simulink model "chirp_rev_detect"  (R2025b)
settings: Solver=FixedStepAuto  StartTime=0.0  StopTime=25  RelTol=1e-3  EnableMultiTasking=on
libraries: dspfdesign x3
settings Model: Creator=Administrator  LastModifiedBy=padhia
settings SolverCC: AlgebraicLoopSolver=TrustRegion  PositivePriorityOrder=on
settings OptimizationCC: EnhancedBackFolding=on  PassReuseOutputArgsAs=Individual arguments  ZeroExternalMemoryAtStartup=off  ZeroInternalMemoryAtStartup=off  MaxStackSize=200000  OptimizeBlockOrder=speed  DifferentSizesBufferReuse=on  OptimizationCustomize=off  EfficientTunableParamExpr=on
settings DebuggingCC: ParameterTunabilityLossMsg=error  UnconnectedInputMsg=warning  UnconnectedOutputMsg=warning  UnconnectedLineMsg=warning
settings HardwareCC: ProdBitPerPointer=32.0  ProdBitPerSizeT=32.0  ProdBitPerPtrDiffT=32.0  ProdLargestAtomicInteger=Long  ProdLargestAtomicFloat=Double  ProdWordSize=32.0  ProdLongLongMode=on  ProdHWDeviceType=ARM Compatible->ARM Cortex-A (32-bit)
settings ModelReferenceCC: EnableRefExpFcnMdlSchedulingChecks=on
settings RTWCC: SystemTargetFile=ert.tlc  GenCodeOnly=on  TemplateMakefile=ert_default_tmf  RTWVerbose=off  Toolchain=GNU GCC Embedded Linux  BuildConfiguration=Faster Runs  IncludeHyperlinkInReport=on  GPUComputeCapability=3.5  Description=Embedded Coder
settings CodeAppCC: ForceParamTrailComments=on  IgnoreCustomStorageClasses=off  OperatorAnnotations=on  SimulinkDataObjDesc=on  SFDataObjDesc=on  InsertBlockDesc=on
settings ERTTargetCC: InlinedParameterPlacement=Hierarchical  ERTCustomFileTemplate=example_file_process.tlc  DynamicArrayContainerType=coder::array  SupportVariableSizeSignals=on

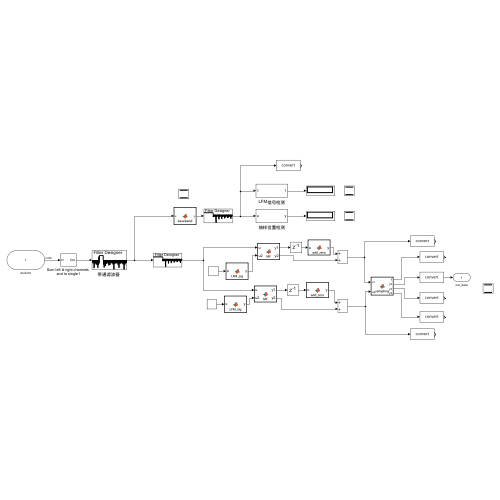
[thumbnail: Simulink's stored preview of the top-level diagram]
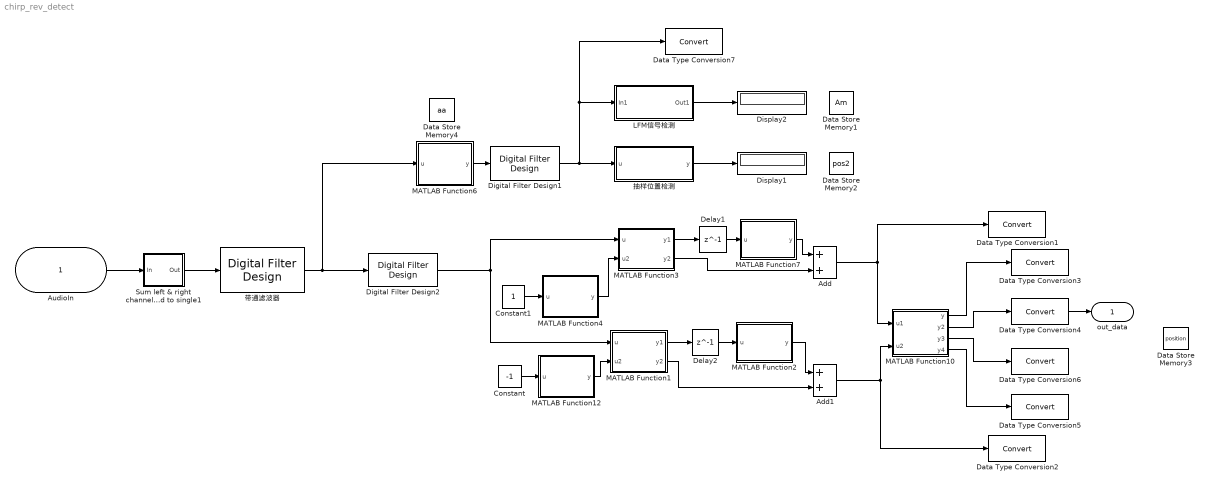
== system chirp_rev_detect ==
  AudioIn : Inport  OutDataTypeStr=int16  PortDimensions=[800 2]  SampleTime=0.1
  Add : Sum
  Add1 : Sum
  Constant : Constant  Value=-1
  Constant1 : Constant
  Data Store Memory1 : DataStoreMemory  DataStoreName=Am  ReadBeforeWriteMsg=warning  WriteAfterWriteMsg=warning  WriteAfterReadMsg=warning  ShowAdditionalParam=off  OutDataTypeStr=double
  Data Store Memory2 : DataStoreMemory  DataStoreName=pos2  ReadBeforeWriteMsg=warning  WriteAfterWriteMsg=warning  WriteAfterReadMsg=warning  ShowAdditionalParam=off  OutDataTypeStr=double
  Data Store Memory3 : DataStoreMemory  DataStoreName=position  ReadBeforeWriteMsg=warning  WriteAfterWriteMsg=warning  WriteAfterReadMsg=warning  ShowAdditionalParam=off  OutDataTypeStr=double
  Data Store Memory4 : DataStoreMemory  DataStoreName=aa  ReadBeforeWriteMsg=warning  WriteAfterWriteMsg=warning  WriteAfterReadMsg=warning  ShowAdditionalParam=off  OutDataTypeStr=double
  Data Type Conversion{1..7} (7 alike) : DataTypeConversion  SaturateOnIntegerOverflow=off  RndMeth=Floor
  Delay1 : Delay  DelayLength=1  InitialCondition=0
  Delay2 : Delay  DelayLength=1  InitialCondition=0
  Digital Filter Design1 : dspfdesign/Digital Filter Design  mwdsp_browser_bugfix_var=off
  Digital Filter Design2 : dspfdesign/Digital Filter Design  mwdsp_browser_bugfix_var=off
  Display1 : Display
  Display2 : Display
  LFM信号检测 : Subsystem
  MATLAB Function1 : MATLAB Function  TreatAsAtomicUnit=on
  MATLAB Function10 : MATLAB Function  TreatAsAtomicUnit=on
  MATLAB Function12 : MATLAB Function  TreatAsAtomicUnit=on
  MATLAB Function2 : MATLAB Function  TreatAsAtomicUnit=on
  MATLAB Function3 : MATLAB Function  TreatAsAtomicUnit=on
  MATLAB Function4 : MATLAB Function  TreatAsAtomicUnit=on
  MATLAB Function6 : MATLAB Function  TreatAsAtomicUnit=on
  MATLAB Function7 : MATLAB Function  TreatAsAtomicUnit=on
  Sum left & right channels and to single1 : Subsystem
  "带通滤波器 " : dspfdesign/Digital Filter Design  mwdsp_browser_bugfix_var=off
  抽样位置检测 : Subsystem
  out_data : Outport
  wires:
  MATLAB Function3/1(y1) -> Delay1/1
  MATLAB Function4/1(y) -> MATLAB Function3/2(u2)
  Digital Filter Design2/1 -> MATLAB Function3/1(u), MATLAB Function1/1(u)
  Add1/1 -> Data Type Conversion2/1, MATLAB Function10/2(u2)
  MATLAB Function10/1(y) -> Data Type Conversion3/1
  MATLAB Function3/2(y2) -> Add/2
  Constant1/1 -> MATLAB Function4/1(u)
  MATLAB Function10/2(y2) -> Data Type Conversion4/1
  Delay2/1 -> MATLAB Function2/1(u)
  MATLAB Function7/1(y) -> Add/1
  Sum left & right channels and to single1/1(Out) -> "带通滤波器 "/1
  MATLAB Function2/1(y) -> Add1/1
  Add/1 -> Data Type Conversion1/1, MATLAB Function10/1(u1)
  MATLAB Function10/3(y3) -> Data Type Conversion6/1
  MATLAB Function1/1(y1) -> Delay2/1
  Constant/1 -> MATLAB Function12/1(u)
  MATLAB Function12/1(y) -> MATLAB Function1/2(u2)
  Delay1/1 -> MATLAB Function7/1(u)
  MATLAB Function1/2(y2) -> Add1/2
  Digital Filter Design1/1 -> 抽样位置检测/1(u), Data Type Conversion7/1, LFM信号检测/1(In1)
  LFM信号检测/1(Out1) -> Display2/1
  "带通滤波器 "/1 -> Digital Filter Design2/1, MATLAB Function6/1(u)
  MATLAB Function6/1(y) -> Digital Filter Design1/1
  MATLAB Function10/4(y4) -> Data Type Conversion5/1
  抽样位置检测/1(y) -> Display1/1
  AudioIn/1 -> Sum left & right channels and to single1/1(In)
  Data Type Conversion4/1 -> out_data/1

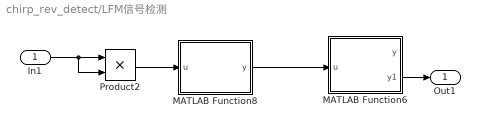
== system chirp_rev_detect/LFM信号检测 ==
  In1 : Inport
  MATLAB Function6 : MATLAB Function  TreatAsAtomicUnit=on
  MATLAB Function8 : MATLAB Function  TreatAsAtomicUnit=on
  Product2 : Product
  Out1 : Outport
  wires:
  Product2/1 -> MATLAB Function8/1(u)
  MATLAB Function8/1(y) -> MATLAB Function6/1(u)
  MATLAB Function6/2(y1) -> Out1/1
  In1/1 -> Product2/2, Product2/1

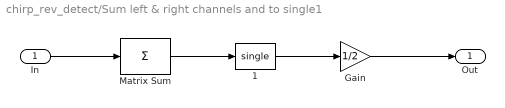
== system chirp_rev_detect/Sum left & right channels and to single1 ==
  In : Inport
  " 1" : DataTypeConversion  OutDataTypeStr=single  SaturateOnIntegerOverflow=off  RndMeth=Floor
  Gain : Gain  Gain=1/2
  Matrix Sum : Sum  Inputs=+  CollapseMode=Specified dimension  CollapseDim=2
  Out : Outport  VectorParamsAs1DForOutWhenUnconnected=off
  wires:
  Gain/1 -> Out/1
  In/1 -> Matrix Sum/1
  Matrix Sum/1 -> " 1"/1
  " 1"/1 -> Gain/1

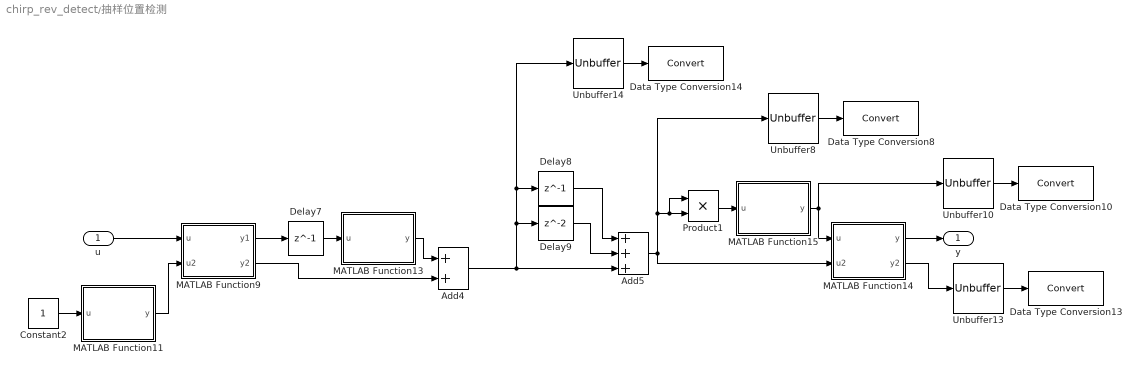
== system chirp_rev_detect/抽样位置检测 ==
  u : Inport
  Add4 : Sum
  Add5 : Sum  Inputs=+++
  Constant2 : Constant
  Data Type Conversion{8,10,13..14} (4 alike) : DataTypeConversion  SaturateOnIntegerOverflow=off  RndMeth=Floor
  Delay7 : Delay  DelayLength=1  InitialCondition=0
  Delay8 : Delay  DelayLength=1  InitialCondition=0
  Delay9 : Delay  InitialCondition=0
  MATLAB Function11 : MATLAB Function  TreatAsAtomicUnit=on
  MATLAB Function13 : MATLAB Function  TreatAsAtomicUnit=on
  MATLAB Function14 : MATLAB Function  TreatAsAtomicUnit=on
  MATLAB Function15 : MATLAB Function  TreatAsAtomicUnit=on
  MATLAB Function9 : MATLAB Function  TreatAsAtomicUnit=on
  Product1 : Product
  Unbuffer{8,10,13..14} (4 alike) : Unbuffer
  y : Outport
  wires:
  Add4/1 -> Unbuffer14/1, Delay8/1, Delay9/1, Add5/3
  MATLAB Function9/2(y2) -> Add4/2
  MATLAB Function11/1(y) -> MATLAB Function9/2(u2)
  Constant2/1 -> MATLAB Function11/1(u)
  Delay7/1 -> MATLAB Function13/1(u)
  MATLAB Function15/1(y) -> Unbuffer10/1, MATLAB Function14/1(u)
  MATLAB Function9/1(y1) -> Delay7/1
  Unbuffer13/1 -> Data Type Conversion13/1
  Delay8/1 -> Add5/1
  MATLAB Function14/2(y2) -> Unbuffer13/1
  Delay9/1 -> Add5/2
  Add5/1 -> MATLAB Function14/2(u2), Unbuffer8/1, Product1/1, Product1/2
  MATLAB Function13/1(y) -> Add4/1
  Unbuffer8/1 -> Data Type Conversion8/1
  Product1/1 -> MATLAB Function15/1(u)
  Unbuffer14/1 -> Data Type Conversion14/1
  Unbuffer10/1 -> Data Type Conversion10/1
  u/1 -> MATLAB Function9/1(u)
  MATLAB Function14/1(y) -> y/1

== matlab function chirp_rev_detect/MATLAB Function12 ==
  data: u input; y output
function y  = LFM_sig(u)
%% miu为1的chrip信号 %%
fs=8000;
T=1e-1;
B=200;                      %信号高频带宽，BT>>1
k=B/T;                      %调频斜率
n=round(T*fs);              %采样点个数
t=linspace(0,T,n);
fc=1000;
miu=u;                      %miu=1时，为Up Chrip信号；miu=-1时，为Down Chrip信号
LFM = exp(j*(2*pi*fc*t + pi*miu*k*t.^2));
%% 时域上的匹配滤波 %%
si=real(LFM);
ht=conj(fliplr(si));
y=ht';

== matlab function chirp_rev_detect/抽样位置检测/MATLAB Function11 ==
  data: u input; y output
function y  = LFM_sig(u)
%% miu为1的chrip信号 %%
fs=8000;
T=1e-1;
B=200;                                       %信号高频带宽，BT>>1
k=B/T;                                       %调频斜率
n=round(T*fs);                               %采样点个数
t=linspace(0,T,n);
% fc=1000;
fc=0;                                        %移植基带
miu=u;                                       %miu=1时，为Up Chrip信号；miu=-1时，为Down Chrip信号
LFM = exp(j*(2*pi*fc*t + pi*miu*k*t.^2));    %线性调频信号复数表达式
%% 时域上的匹配滤波 %%
si=real(LFM);                                %取chrip信号实部
ht=conj(fliplr(si));                         %时域上的匹配滤波：ht=Ks(t0-t)，参考博客https://blog.csdn.net/ccsss22/article/details/108761297
y=ht';

== matlab function chirp_rev_detect/抽样位置检测/MATLAB Function13 ==
  data: u input; y output
function y = add_zero(u)
y=[u;0];

== matlab function chirp_rev_detect/抽样位置检测/MATLAB Function14 ==
  data: u input; y output; pos2 data_store_memory; Am data_store_memory; y2 output; u2 input
function [y,y2] = detect(u,u2)
global pos2
global Am
persistent loc
persistent aa
persistent flag
if isempty(loc)
    loc=0;
end
if isempty(aa)
    aa=0;
end
if isempty(flag)
    flag=0;
end

if Am>0
    if u > 20*Am && u>5*1e3
        loc=loc+1;
    else
        loc=0;
    end

    if loc>3                 %连续3帧数据到来后，flag=1，开始求抽样点
        flag=flag+1;
    end
    if flag==1
        [Y,I]=max(abs(u2));
        if abs(u2(I))>3*1e4
            aa=I;flag=2;
        end
    end
end
% if u(aa)>5*1e3
    pos2=aa;
% end
y2=aa;
y=pos2;

== matlab function chirp_rev_detect/抽样位置检测/MATLAB Function15 ==
  data: u input; y output
function y= sum1(u)
tem1=sum(u)/length(u); %求每帧信号功率
A=sqrt(2*tem1);        %根据公式P=A^2/2求出A
y=A;

== matlab function chirp_rev_detect/抽样位置检测/MATLAB Function9 ==
  data: u input; y1 output; y2 output; u2 input
function [y1,y2] = MF(u,u2)
%% 匹配滤波 %%
temp=conv(u,u2);
y2=temp(1:length(u));  %分成两路输出，其中一路延迟后累加，y2大小为80*1，y2大小为79*1
y1=temp(length(u)+1:end);

== matlab function chirp_rev_detect/MATLAB Function1 ==
  data: u input; y1 output; y2 output; u2 input
function [y1,y2] = MF(u,u2)
%% 匹配滤波 %%
temp=conv(u,u2);
y2=temp(1:length(u));  %分成两路输出，其中一路延迟后累加，y2大小为80*1，y2大小为79*1
y1=temp(length(u)+1:end);

== matlab function chirp_rev_detect/MATLAB Function2 ==
  data: u input; y output
function y = add_zero(u)
y=[u;0];

== matlab function chirp_rev_detect/MATLAB Function3 ==
  data: u input; y1 output; y2 output; u2 input
function [y1,y2] = MF(u,u2)
%% 匹配滤波 %%
temp=conv(u,u2);
y2=temp(1:length(u));  %分成两路输出，其中一路延迟后累加，y2大小为80*1，y2大小为79*1
y1=temp(length(u)+1:end);

== matlab function chirp_rev_detect/MATLAB Function4 ==
  data: u input; y output
function y  = LFM_sig(u)
%% miu为1的chrip信号 %%
fs=8000;
T=1e-1;
B=200;                      %信号高频带宽，BT>>1
k=B/T;                      %调频斜率
n=round(T*fs);              %采样点个数
t=linspace(0,T,n);
fc=1000;
miu=u;                      %miu=1时，为Up Chrip信号；miu=-1时，为Down Chrip信号
LFM = exp(j*(2*pi*fc*t + pi*miu*k*t.^2)); 
%% 时域上的匹配滤波 %%
si=real(LFM);
ht=conj(fliplr(si)); 
y=ht';

== matlab function chirp_rev_detect/MATLAB Function6 ==
  data: u input; y output; aa data_store_memory
function y= baseband(u)
global aa

fs=8000;                    %采样率
T=1e-1;                     %0.1  
n=round(T*fs);              %采样点个数，800
t=linspace(0,T,n);          %0-T之间n等分
fc=1000;
u1=cos(2*pi*fc*(t+aa*T));
ht=u1';
baseband=u.*(ht);
aa=aa+1;
y=baseband;

== matlab function chirp_rev_detect/MATLAB Function7 ==
  data: u input; y output
function y = add_zero(u)
y=[u;0];

== matlab function chirp_rev_detect/LFM信号检测/MATLAB Function6 ==
  data: u input; y output; Am data_store_memory; y1 output
function [ y, y1]= sum2(u)
persistent loc
persistent flag
global Am

if isempty(loc)
    loc=0;
end
if isempty(flag)
    flag=0;
end

 if u > 10                 %输出值为A 
    loc=loc+1;
else
    loc=0;
end

if loc>10                 %连续3帧数据到来后，flag=1，开始求Am
    flag=flag+1;
    y=u;
else
    y=single(0);
end

if flag==1
    u=double(u);
    Am=u;
end
y1=Am;

== matlab function chirp_rev_detect/LFM信号检测/MATLAB Function8 ==
  data: u input; y output
function y= sum1(u)
tem1=sum(u)/length(u); %求每帧信号功率
A=sqrt(2*tem1);        %根据公式P=A^2/2求出A
y=A;

== matlab function chirp_rev_detect/MATLAB Function10 ==
  data: u1 input; y output; u2 input; y2 output; y3 output; Am data_store_memory; position data_store_memory; pos2 data_store_memory; y4 output
function [ y , y2, y3, y4]  = sampling(u1 , u2)    %u1为miu=1匹配滤波输出，u2为miu=-1匹配滤波输出
global pos2
global Am
global position
persistent position11
if isempty(position11)
    position11=0;
end

if Am>0        
    position=pos2; 
end

if position>0        
    range=50;
    max1=max(abs(u1(position-range:position+range)));   %误差补足
    max2=max(abs(u2(position-range:position+range)));
    if max1 > max2
        y2=single(1);
    else
        y2=single(-1);
    end
    y3=max1;
    y4=max2;
else
    y2=single(0);
    y3=single(0);
    y4=single(0);
end
y=position;
